simulink model "sampleModel1000"  (R2022a)
settings: Solver=VariableStepAuto  StartTime=0.0  StopTime=10.0  RelTol=1e-3
undefined symbols (not defined in the file): DiscIntNeverNeededParam, magnitude, Newton, Raphson
libraries: simulink x216, slpidlib x76
(part 1 of 10)
settings Model: Creator=TSMC  LastModifiedBy=TSMC

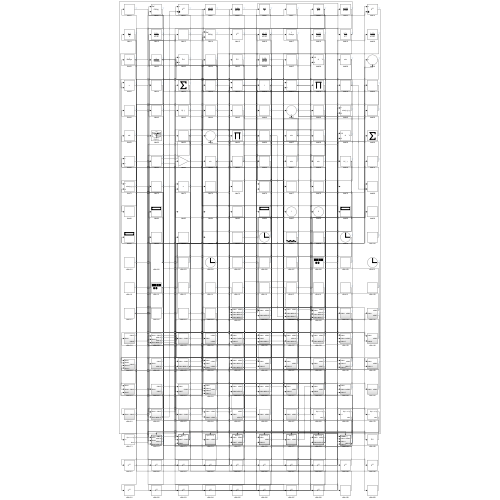
[thumbnail: Simulink's stored preview of the top-level diagram]
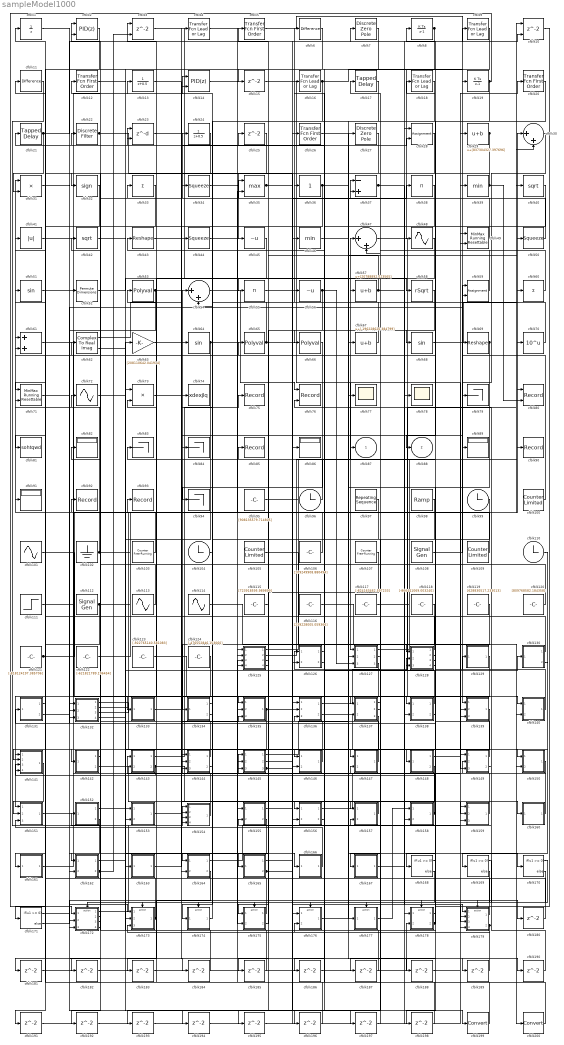
== system sampleModel1000 ==
  cfblk1 : UnitDelay  HasFrameUpgradeWarning=on
  cfblk10 : Delay  ShowEnablePort=on  SampleTime=1
      settings: InputPortMap=u0,e6
  cfblk100 : simulink/Sources/Counter Limited  uplimit=[967.000000]  tsamp=-1
  cfblk101 : Sin  Amplitude=[773063809.845792]  Bias=[655952196.754793]  SampleTime=0
  cfblk102 : Ground
  cfblk103 : simulink/Sources/Counter Free-Running  NumBits=[40.000000]  tsamp=-1
  cfblk{96,99,104,110} (4 alike) : Clock
  cfblk105 : simulink/Sources/Counter Limited  uplimit=[424.000000]  tsamp=-1
  cfblk106 : Constant  Value=[109249908.880494]  SampleTime=1
  cfblk107 : simulink/Sources/Counter Free-Running  NumBits=[50.000000]  tsamp=-1
  cfblk108 : SignalGenerator  WaveForm=sawtooth  Amplitude=[13452965.710921]
  cfblk109 : simulink/Sources/Counter Limited  uplimit=[559.000000]  tsamp=-1
  cfblk11 : simulink/Discrete/Difference  ICPrevInput=0.0  OutMin=[]  OutMax=[]  OutDataTypeStr=Inherit: Inherit via back propagation  OutDataType=fixdt(1, 16)  OutScaling=2^-10  DoSatur=off
  cfblk111 : Step  Time=[14.000000]  Before=[-58060012.443622]  After=[794614404.214897]  SampleTime=0
  cfblk112 : SignalGenerator  WaveForm=sawtooth  Amplitude=[-762282920.604162]  Units=rad/sec
  cfblk113 : Sin  Amplitude=[-356034610.083544]  Bias=[-701710230.192612]  SampleTime=0
  cfblk114 : Sin  Amplitude=[643616227.211529]  Bias=[3557649.516432]  SampleTime=0
  cfblk115 : Constant  Value=[723918595.989899]  SampleTime=1
  cfblk116 : Constant  Value=[239228005.059366]  SampleTime=1
  cfblk117 : Constant  Value=[-824163462.597233]  SampleTime=1
  cfblk118 : Constant  Value=[-866441069.003240]  SampleTime=1
  cfblk119 : Constant  Value=[628830517.233013]  SampleTime=1
  cfblk{5,12,20,26} (4 alike) : simulink/Discrete/Transfer Fcn First Order  PoleZ=0.95  ICPrevOutput=0.0  DoSatur=off
  cfblk120 : Constant  Value=[809768582.184358]  SampleTime=1
  cfblk121 : Constant  Value=[-818124197.385706]  SampleTime=1
  cfblk122 : Constant  Value=[-621821789.196454]  SampleTime=1
  cfblk123 : Constant  Value=[-922765140.581083]  SampleTime=1
  cfblk124 : Constant  Value=[-476552846.153060]  SampleTime=1
  cfblk125 : Subsystem
  cfblk126 : Subsystem
  cfblk127 : Subsystem
  cfblk128 : Subsystem
  cfblk129 : Subsystem
  cfblk13 : DiscreteTransferFcn  SampleTime=1
  cfblk130 : Subsystem
  cfblk131 : Subsystem
  cfblk132 : Subsystem
  cfblk133 : Subsystem
  cfblk134 : Subsystem
  cfblk135 : Subsystem
  cfblk136 : Subsystem
  cfblk137 : Subsystem
  cfblk138 : Subsystem
  cfblk139 : Subsystem
  cfblk14 : slpidlib/PID Controller (2DOF)  Controller=PID  Form=Parallel  TimeDomain=Discrete-time  UseExternalTs=off  SampleTime=1  IntegratorMethod=Forward Euler  FilterMethod=Forward Euler  ControllerParametersSource=internal  P=1  I=1  UseKiTs=off  D=0  N=100  UseFilter=on  b=1  c=1  TunerSelectOption=Transfer Function Based (PID Tuner App)  InitialConditionSource=internal  InitialConditionForIntegrator=0  InitialConditionForFilter=0  DifferentiatorICPrevScaledInput=0  ExternalReset=none  TrackingMode=off  Kt=1  LimitOutput=off  SatLimitsSource=internal  UpperSaturationLimit=inf  LowerSaturationLimit=-inf  LinearizeAsGain=off  AntiWindupMode=none  Kb=1  POutMin=[]  POutMax=[]  IOutMin=[]  IOutMax=[]  DOutMin=[]  DOutMax=[]  NOutMin=[]  NOutMax=[]  bOutMin=[]  bOutMax=[]  cOutMin=[]  cOutMax=[]  SumOutMin=[]  SumOutMax=[]  SaturationOutMin=[]  SaturationOutMax=[]  PParamMin=[]  PParamMax=[]  IParamMin=[]  IParamMax=[]  DParamMin=[]  DParamMax=[]  NParamMin=[]  NParamMax=[]  bParamMin=[]  bParamMax=[]  cParamMin=[]  cParamMax=[]  KbParamMin=[]  KbParamMax=[]  KtParamMin=[]  KtParamMax=[]  KbOutMin=[]  KbOutMax=[]  KtOutMin=[]  KtOutMax=[]  IntegratorOutMin=[]  IntegratorOutMax=[]  FilterOutMin=[]  FilterOutMax=[]  SumI1OutMin=[]  SumI1OutMax=[]  SumI2OutMin=[]  SumI2OutMax=[]  SumI3OutMin=[]  SumI3OutMax=[]  SumI4OutMin=[]  SumI4OutMax=[]  SumDOutMin=[]  SumDOutMax=[]  Sum1OutMin=[]  Sum1OutMax=[]  Sum2OutMin=[]  Sum2OutMax=[]  Sum3OutMin=[]  Sum3OutMax=[]  DifferentiatorOutMin=[]  DifferentiatorOutMax=[]  FilterDiffOutCoefMin=[]  FilterDiffOutCoefMax=[]  ReciprocalOutMin=[]  ReciprocalOutMax=[]  SumDenOutMin=[]  SumDenOutMax=[]  SumNumOutMin=[]  SumNumOutMax=[]  DivideOutMin=[]  DivideOutMax=[]  UdiffTsProdOutMin=[]  UdiffTsProdOutMax=[]  NTsProdOutMin=[]  NTsProdOutMax=[]  UintegralTsProdOutMin=[]  UintegralTsProdOutMax=[]  UngainTsProdOutMin=[]  UngainTsProdOutMax=[]  IntegratorContinuousStateAttributes=''  IntegratorStateMustResolveToSignalObject=off  IntegratorRTWStateStorageClass=Auto  FilterContinuousStateAttributes=''  FilterStateMustResolveToSignalObject=off  FilterRTWStateStorageClass=Auto  ParallelPVariant=InternalParameters  IdealPVariant=Disabled  IVariant=InternalParameters  DVariant=InternalParameters  bVariant=InternalParameters  cVariant=InternalParameters  IntegratorVariant=Discrete  SatVariant=Disabled  AWVariant=Passthrough  PCopyVariant=Disabled  TRVariant=Disabled  FdbkBlocksVariant=Forward  IdealPFdbkVariant=Disabled  SatFdbkVariant=Disabled  DerivativeFilterVariant=ForwardEulerFilter  NVariant=InternalParameters  NCopyVariant=Disabled  FilterICVariant=InternalICsFilter  IntegratorICVariant=InternalICs  ExternalResetVariant=Disabled  TRSumVariant=Passthrough  SumFdbkVariant=Disabled  SumVariant=Sum_PID  TsampFilterVariant=InternalTs  TsampNgainVariant=Passthrough  TsampIntegralVariant=Passthrough  ExternalSaturationOutDataTypeStr=Inherit: Same as second input
      settings: SourceProductBaseCode=SL
  cfblk140 : Subsystem
  cfblk141 : Subsystem
  cfblk142 : Subsystem
  cfblk143 : Subsystem
  cfblk144 : Subsystem
  cfblk145 : Subsystem
  cfblk146 : Subsystem
  cfblk147 : Subsystem
  cfblk148 : Subsystem
  cfblk149 : Subsystem
  cfblk{15,25,180..198} (21 alike) : Delay  SampleTime=1
  cfblk150 : Subsystem
  cfblk151 : Subsystem
  cfblk152 : Subsystem
  cfblk153 : Subsystem
  cfblk154 : Subsystem
  cfblk155 : Subsystem
  cfblk156 : Subsystem
  cfblk157 : Subsystem
  cfblk158 : Subsystem
  cfblk159 : Subsystem
  cfblk{4,9,16,18} (4 alike) : simulink/Discrete/Transfer Fcn Lead or Lag  PoleZ=0.95  ZeroZ=0.75  ICPrevOutput=0.0  ICPrevInput=0.0  DoSatur=off
      settings: SourceProductBaseCode=SL
  cfblk160 : Subsystem
  cfblk161 : Subsystem
  cfblk162 : Subsystem
  cfblk163 : Subsystem
  cfblk164 : Subsystem
  cfblk165 : Subsystem
  cfblk166 : Subsystem
  cfblk167 : Subsystem
  cfblk{168..171} (4 alike) : If  IfExpression=u1 >= 0  SampleTime=1
  cfblk17 : simulink/Discrete/Tapped Delay  vinit=0.0  samptime=-1  NumDelays=1  DelayOrder=Oldest  includeCurrent=off
  cfblk172 : Subsystem  TreatAsAtomicUnit=on
  cfblk173 : Subsystem  TreatAsAtomicUnit=on
  cfblk174 : Subsystem  TreatAsAtomicUnit=on
  cfblk175 : Subsystem  TreatAsAtomicUnit=on
  cfblk176 : Subsystem  TreatAsAtomicUnit=on
  cfblk177 : Subsystem  TreatAsAtomicUnit=on
  cfblk178 : Subsystem  TreatAsAtomicUnit=on
  cfblk179 : Subsystem  TreatAsAtomicUnit=on
  cfblk19 : DiscreteIntegrator  ICPrevOutput=DiscIntNeverNeededParam  ICPrevScaledInput=DiscIntNeverNeededParam
  cfblk199 : DataTypeConversion  SaturateOnIntegerOverflow=off  RndMeth=Floor
  cfblk2 : slpidlib/PID Controller (2DOF)  Controller=PID  Form=Parallel  TimeDomain=Discrete-time  UseExternalTs=off  SampleTime=1  IntegratorMethod=Forward Euler  FilterMethod=Forward Euler  ControllerParametersSource=internal  P=1  I=1  UseKiTs=off  D=0  N=100  UseFilter=on  b=1  c=1  TunerSelectOption=Transfer Function Based (PID Tuner App)  InitialConditionSource=internal  InitialConditionForIntegrator=0  InitialConditionForFilter=0  DifferentiatorICPrevScaledInput=0  ExternalReset=none  TrackingMode=off  Kt=1  LimitOutput=off  SatLimitsSource=internal  UpperSaturationLimit=inf  LowerSaturationLimit=-inf  LinearizeAsGain=off  AntiWindupMode=none  Kb=1  POutMin=[]  POutMax=[]  IOutMin=[]  IOutMax=[]  DOutMin=[]  DOutMax=[]  NOutMin=[]  NOutMax=[]  bOutMin=[]  bOutMax=[]  cOutMin=[]  cOutMax=[]  SumOutMin=[]  SumOutMax=[]  SaturationOutMin=[]  SaturationOutMax=[]  PParamMin=[]  PParamMax=[]  IParamMin=[]  IParamMax=[]  DParamMin=[]  DParamMax=[]  NParamMin=[]  NParamMax=[]  bParamMin=[]  bParamMax=[]  cParamMin=[]  cParamMax=[]  KbParamMin=[]  KbParamMax=[]  KtParamMin=[]  KtParamMax=[]  KbOutMin=[]  KbOutMax=[]  KtOutMin=[]  KtOutMax=[]  IntegratorOutMin=[]  IntegratorOutMax=[]  FilterOutMin=[]  FilterOutMax=[]  SumI1OutMin=[]  SumI1OutMax=[]  SumI2OutMin=[]  SumI2OutMax=[]  SumI3OutMin=[]  SumI3OutMax=[]  SumI4OutMin=[]  SumI4OutMax=[]  SumDOutMin=[]  SumDOutMax=[]  Sum1OutMin=[]  Sum1OutMax=[]  Sum2OutMin=[]  Sum2OutMax=[]  Sum3OutMin=[]  Sum3OutMax=[]  DifferentiatorOutMin=[]  DifferentiatorOutMax=[]  FilterDiffOutCoefMin=[]  FilterDiffOutCoefMax=[]  ReciprocalOutMin=[]  ReciprocalOutMax=[]  SumDenOutMin=[]  SumDenOutMax=[]  SumNumOutMin=[]  SumNumOutMax=[]  DivideOutMin=[]  DivideOutMax=[]  UdiffTsProdOutMin=[]  UdiffTsProdOutMax=[]  NTsProdOutMin=[]  NTsProdOutMax=[]  UintegralTsProdOutMin=[]  UintegralTsProdOutMax=[]  UngainTsProdOutMin=[]  UngainTsProdOutMax=[]  IntegratorContinuousStateAttributes=''  IntegratorStateMustResolveToSignalObject=off  IntegratorRTWStateStorageClass=Auto  FilterContinuousStateAttributes=''  FilterStateMustResolveToSignalObject=off  FilterRTWStateStorageClass=Auto  ParallelPVariant=InternalParameters  IdealPVariant=Disabled  IVariant=InternalParameters  DVariant=InternalParameters  bVariant=InternalParameters  cVariant=InternalParameters  IntegratorVariant=Discrete  SatVariant=Disabled  AWVariant=Passthrough  PCopyVariant=Disabled  TRVariant=Disabled  FdbkBlocksVariant=Forward  IdealPFdbkVariant=Disabled  SatFdbkVariant=Disabled  DerivativeFilterVariant=ForwardEulerFilter  NVariant=InternalParameters  NCopyVariant=Disabled  FilterICVariant=InternalICsFilter  IntegratorICVariant=InternalICs  ExternalResetVariant=Disabled  TRSumVariant=Passthrough  SumFdbkVariant=Disabled  SumVariant=Sum_PID  TsampFilterVariant=InternalTs  TsampNgainVariant=Passthrough  TsampIntegralVariant=Passthrough  ExternalSaturationOutDataTypeStr=Inherit: Same as second input
      settings: SourceProductBaseCode=SL
  cfblk200 : DataTypeConversion  SaturateOnIntegerOverflow=off  RndMeth=Floor
  cfblk21 : simulink/Discrete/Tapped Delay  vinit=0.0  samptime=-1  NumDelays=1  DelayOrder=Oldest  includeCurrent=off
  cfblk22 : DiscreteFilter  SampleTime=1
  cfblk23 : Delay  DelayLengthSource=Input port  SampleTime=1
      settings: InputPortMap=u0,p1
  cfblk24 : DiscreteTransferFcn  SampleTime=1
  cfblk27 : DiscreteZeroPole  Poles=[0 0.5]  Gain=1
  cfblk28 : Assignment  DiagnosticForDimensions=Warning  IndexOptions=Index vector (dialog)  Indices=1  OutputSizes=1
  cfblk29 : Bias  Bias=[837304327.397696]  SaturateOnIntegerOverflow=off
  cfblk3 : Delay  ShowEnablePort=on  SampleTime=1
      settings: InputPortMap=u0,e6
  cfblk30 : Sum  Inputs=|++
  cfblk31 : Product
  cfblk32 : Signum
  cfblk33 : Sum  Inputs=+
  cfblk34 : Squeeze
  cfblk35 : MinMax  Function=max  Inputs=2
  cfblk36 : simulink/Math Operations/Slider Gain  gain=1  low=0  high=2
  cfblk37 : Sum  Inputs=-+
  cfblk38 : Product  Inputs=*
  cfblk39 : MinMax
  cfblk40 : Sqrt
  cfblk41 : Abs  SaturateOnIntegerOverflow=off
  cfblk42 : Sqrt
  cfblk43 : Reshape
  cfblk44 : Squeeze
  cfblk45 : UnaryMinus
  cfblk46 : MinMax
  cfblk47 : Sum  Inputs=|++
  cfblk48 : Sin  TimeSource=Use external signal  SampleTime=0
  cfblk49 : simulink/Math Operations/MinMax Running Resettable  Function=min  vinit=0.0
  cfblk50 : Squeeze
  cfblk51 : Trigonometry
  cfblk52 : PermuteDimensions
  cfblk53 : Polyval  Coefs=[ +2.081618890e-019, -1.441693666e-014, +4.719686976e-010, -8.536869453e-006, +1.621573104e-001, -8.087801117e+001 ]
  cfblk54 : Sum  Inputs=|++
  cfblk55 : Product  Inputs=*
  cfblk56 : UnaryMinus
  cfblk57 : Bias  Bias=[20788892.023565]  SaturateOnIntegerOverflow=off
  cfblk58 : Sqrt  Operator=rSqrt  AlgorithmType=Newton-Raphson
  cfblk59 : Assignment  DiagnosticForDimensions=Warning  IndexOptions=Index vector (dialog)  Indices=1  OutputSizes=1
  cfblk6 : simulink/Discrete/Difference  ICPrevInput=0.0  OutMin=[]  OutMax=[]  OutDataTypeStr=Inherit: Inherit via back propagation  OutDataType=fixdt(1, 16)  OutScaling=2^-10  DoSatur=off
  cfblk60 : Sum  Inputs=+
  cfblk61 : Sum
  cfblk62 : ComplexToRealImag
  cfblk63 : Gain  Gain=[208110642.041914]
  cfblk64 : Trigonometry
  cfblk65 : Polyval  Coefs=[ +2.081618890e-019, -1.441693666e-014, +4.719686976e-010, -8.536869453e-006, +1.621573104e-001, -8.087801117e+001 ]
  cfblk66 : Polyval  Coefs=[ +2.081618890e-019, -1.441693666e-014, +4.719686976e-010, -8.536869453e-006, +1.621573104e-001, -8.087801117e+001 ]
  cfblk67 : Bias  Bias=[-196228620.384799]  SaturateOnIntegerOverflow=off
  cfblk68 : Trigonometry
  cfblk69 : Reshape
  cfblk7 : DiscreteZeroPole  Poles=[0 0.5]  Gain=1
  cfblk70 : Math  Operator=10^u
  cfblk71 : simulink/Math Operations/MinMax Running Resettable  Function=min  vinit=0.0
  cfblk72 : Sin  TimeSource=Use external signal  SampleTime=0
  cfblk73 : Product  Inputs=**
  cfblk74 : ToWorkspace  VariableName=xdexjlq  SaveFormat=Timeseries  SampleTime=-1
  cfblk75 : Record  FileSettingsInternal="{\"entries\":[{\"content\":{\"excelSettings\":{\"content\":{},\"type\":\"Streamout.ExcelSettings\"}},\"type\":\"Streamout.FileSettingStorage\",\"uuid\":\"93119369-c950-46ca-a22c-1d32b41a04c2\"}],\"packageUris\":[\"http://schema.mathworks.com/mf0/streamout_blocks/R2020a\"],\"version\":\"1.0\"}"  SignalsInternal="{\"entries\":[{\"content\":{\"signals\":[]},\"type\":\"RecordBlkView.InputSignals\",\"uuid\":\"8868a1fd-9bce-4a45-8f3b-298cfc814564\"}],\"packageUris\":[\"http://schema.mathworks.com/mf0/streamout_blocks/R2020a\"],\"version\":\"1.0\"}"  VisualizationBindings="{\"sparklinesplugin\":{\"info\":[{\"bindingParametersList\":[],\"subplotID\":1}]}}"
  cfblk76 : Record  FileSettingsInternal="{\"entries\":[{\"content\":{\"excelSettings\":{\"content\":{},\"type\":\"Streamout.ExcelSettings\"}},\"type\":\"Streamout.FileSettingStorage\",\"uuid\":\"a03253ba-281f-4ced-abad-5bfd2517a59d\"}],\"packageUris\":[\"http://schema.mathworks.com/mf0/streamout_blocks/R2020a\"],\"version\":\"1.0\"}"  Layout=[1 1]  SignalsInternal="{\"entries\":[{\"content\":{\"signals\":[{\"content\":{\"blockPath\":[\"sampleModel93/cfblk76\"],\"channel\":[],\"dimensions\":[1],\"domain\":\"sampleModel93/cfblk76\",\"lineColor\":\"#a2142f\",\"plots\":[1],\"port\":1,\"sid\":[],\"signalID\":93159,\"signalName\":\"XY Graph:1\"},\"type\":\"RecordBlkView.Signal\",\"uuid\":\"edc37d75-abdc-4082-bde9-98d4d700ed05\"},{\"content\":{\"blockPath\":[\"sampleModel93/cfblk76\"],\"channel\":[],\"dimensions\":[1],\"domain\":\"sampleModel93/cfblk76\",\"lineColor\":\"#139fff\",\"plots\":[1],\"port\":2,\"sid\":[],\"signalID\":93162,\"signalName\":\"XY Graph:2\"},\"type\":\"RecordBlkView.Signal\",\"uuid\":\"72f55811-d401-47ba-bcf8-176263eeb075\"}]},\"type\":\"RecordBlkView.InputSignals\",\"uuid\":\"5a81d43f-68da-4077-b013-bac875f31b79\"}],\"packageUris\":[\"http://schema.mathworks.com/mf0/streamout_blocks/R2020a\"],\"version\":\"1.0\"}"  VisualizationBindings="{\"xyplotplugin\":{\"info\":[{\"series\":[{\"bindingParametersList\":[{\"parameter\":\"X-Axis\",\"signalID\":93159,\"signalName\":\"XY Graph:1\"},{\"parameter\":\"Y-Axis\",\"signalID\":93162,\"signalName\":\"XY Graph:2\"}],\"seriesID\":38366}],\"subplotID\":1}]}}"  CompatibilityTag=XY
  cfblk77 : Scope
  cfblk78 : Scope
  cfblk{79,83..84,94} (4 alike) : Terminator
  cfblk8 : DiscreteIntegrator  ICPrevOutput=DiscIntNeverNeededParam  ICPrevScaledInput=DiscIntNeverNeededParam
  cfblk80 : Record  FileSettingsInternal="{\"entries\":[{\"content\":{\"excelSettings\":{\"content\":{},\"type\":\"Streamout.ExcelSettings\"}},\"type\":\"Streamout.FileSettingStorage\",\"uuid\":\"2507d3ea-2c9f-47b8-9c6a-10834b2444f5\"}],\"packageUris\":[\"http://schema.mathworks.com/mf0/streamout_blocks/R2020a\"],\"version\":\"1.0\"}"  Layout=[1 1]  SignalsInternal="{\"entries\":[{\"content\":{\"signals\":[{\"content\":{\"blockPath\":[\"sampleModel93/cfblk80\"],\"channel\":[],\"dimensions\":[1],\"domain\":\"sampleModel93/cfblk80\",\"lineColor\":\"#a2142f\",\"plots\":[1],\"port\":1,\"sid\":[],\"signalID\":93167,\"signalName\":\"XY Graph:1\"},\"type\":\"RecordBlkView.Signal\",\"uuid\":\"5814ea94-654b-43ff-b425-7d5855ec870a\"},{\"content\":{\"blockPath\":[\"sampleModel93/cfblk80\"],\"channel\":[],\"dimensions\":[1],\"domain\":\"sampleModel93/cfblk80\",\"lineColor\":\"#139fff\",\"plots\":[1],\"port\":2,\"sid\":[],\"signalID\":93170,\"signalName\":\"XY Graph:2\"},\"type\":\"RecordBlkView.Signal\",\"uuid\":\"afd25cc8-4550-43db-8d86-e57050363295\"}]},\"type\":\"RecordBlkView.InputSignals\",\"uuid\":\"2447f943-610b-4a01-b7b9-18fff63071f0\"}],\"packageUris\":[\"http://schema.mathworks.com/mf0/streamout_blocks/R2020a\"],\"version\":\"1.0\"}"  VisualizationBindings="{\"xyplotplugin\":{\"info\":[{\"series\":[{\"bindingParametersList\":[{\"parameter\":\"X-Axis\",\"signalID\":93167,\"signalName\":\"XY Graph:1\"},{\"parameter\":\"Y-Axis\",\"signalID\":93170,\"signalName\":\"XY Graph:2\"}],\"seriesID\":65284}],\"subplotID\":1}]}}"  CompatibilityTag=XY
  cfblk81 : ToWorkspace  VariableName=sohtqwd  SaveFormat=Timeseries  SampleTime=-1
  cfblk{82,86,89,91} (4 alike) : Display
  cfblk85 : Record  FileSettingsInternal="{\"entries\":[{\"content\":{\"excelSettings\":{\"content\":{},\"type\":\"Streamout.ExcelSettings\"}},\"type\":\"Streamout.FileSettingStorage\",\"uuid\":\"56e11c23-7fef-42fd-95e6-2b1f2738764b\"}],\"packageUris\":[\"http://schema.mathworks.com/mf0/streamout_blocks/R2020a\"],\"version\":\"1.0\"}"  SignalsInternal="{\"entries\":[{\"content\":{\"signals\":[]},\"type\":\"RecordBlkView.InputSignals\",\"uuid\":\"a01aa0e3-d666-47db-b4e9-c308bb60c8cd\"}],\"packageUris\":[\"http://schema.mathworks.com/mf0/streamout_blocks/R2020a\"],\"version\":\"1.0\"}"  VisualizationBindings="{\"sparklinesplugin\":{\"info\":[{\"bindingParametersList\":[],\"subplotID\":1}]}}"
  cfblk90 : Record  FileSettingsInternal="{\"entries\":[{\"content\":{\"excelSettings\":{\"content\":{},\"type\":\"Streamout.ExcelSettings\"}},\"type\":\"Streamout.FileSettingStorage\",\"uuid\":\"6dada1e4-55e1-4f5a-970b-daff20d2999b\"}],\"packageUris\":[\"http://schema.mathworks.com/mf0/streamout_blocks/R2020a\"],\"version\":\"1.0\"}"  SignalsInternal="{\"entries\":[{\"content\":{\"signals\":[]},\"type\":\"RecordBlkView.InputSignals\",\"uuid\":\"89ee935f-d475-4a10-a7b9-b698c62ff7ff\"}],\"packageUris\":[\"http://schema.mathworks.com/mf0/streamout_blocks/R2020a\"],\"version\":\"1.0\"}"  VisualizationBindings="{\"sparklinesplugin\":{\"info\":[{\"bindingParametersList\":[],\"subplotID\":1}]}}"
  cfblk92 : Record  FileSettingsInternal="{\"entries\":[{\"content\":{\"excelSettings\":{\"content\":{},\"type\":\"Streamout.ExcelSettings\"}},\"type\":\"Streamout.FileSettingStorage\",\"uuid\":\"1238a7f8-d0eb-4180-8fbc-9d1406293420\"}],\"packageUris\":[\"http://schema.mathworks.com/mf0/streamout_blocks/R2020a\"],\"version\":\"1.0\"}"  SignalsInternal="{\"entries\":[{\"content\":{\"signals\":[]},\"type\":\"RecordBlkView.InputSignals\",\"uuid\":\"67d9e696-d9a1-4a8c-bdff-202bc9e338b2\"}],\"packageUris\":[\"http://schema.mathworks.com/mf0/streamout_blocks/R2020a\"],\"version\":\"1.0\"}"  VisualizationBindings="{\"sparklinesplugin\":{\"info\":[{\"bindingParametersList\":[],\"subplotID\":1}]}}"
  cfblk93 : Record  FileSettingsInternal="{\"entries\":[{\"content\":{\"excelSettings\":{\"content\":{},\"type\":\"Streamout.ExcelSettings\"}},\"type\":\"Streamout.FileSettingStorage\",\"uuid\":\"aa34f245-15e1-43bc-9a71-911d6946ae5d\"}],\"packageUris\":[\"http://schema.mathworks.com/mf0/streamout_blocks/R2020a\"],\"version\":\"1.0\"}"  SignalsInternal="{\"entries\":[{\"content\":{\"signals\":[]},\"type\":\"RecordBlkView.InputSignals\",\"uuid\":\"ca37f52f-a70f-4701-97d8-d5f8771f9d64\"}],\"packageUris\":[\"http://schema.mathworks.com/mf0/streamout_blocks/R2020a\"],\"version\":\"1.0\"}"  VisualizationBindings="{\"sparklinesplugin\":{\"info\":[{\"bindingParametersList\":[],\"subplotID\":1}]}}"
  cfblk95 : Constant  Value=[908135579.714805]  SampleTime=1
  cfblk97 : simulink/Sources/Repeating Sequence  rep_seq_t=[0 2]  rep_seq_y=[-687576342.069887, -842837087.753460]
  cfblk98 : simulink/Sources/Ramp  slope=[9655.940624]  start=[7.462579]  InitialOutput=[164286.432443]
  cfblk87 : Outport
  cfblk88 : Outport  Port=2
  wires:
  cfblk124/1 -> cfblk151/1(cfblk1)
  cfblk66/1 -> cfblk174/1(cfblk1)
  cfblk54/1 -> cfblk76/1
  cfblk154/1(cfblk2) -> cfblk54/1
  cfblk58/1 -> cfblk135/1(cfblk1)
  cfblk3/1 -> cfblk86/1
  cfblk6/1 -> cfblk15/1
  cfblk11/1 -> cfblk154/1(cfblk1)
  cfblk151/1(cfblk2) -> cfblk14/1
  cfblk5/1 -> cfblk139/1(cfblk1)
  cfblk70/1 -> cfblk21/1
  cfblk47/1 -> cfblk140/1(cfblk1)
  cfblk177/1(cfblk2) -> cfblk158/1(cfblk1)
  cfblk108/1 -> cfblk59/1
  cfblk49/1 -> cfblk24/1
  cfblk25/1 -> cfblk45/1
  cfblk125/1(cfblk2) -> cfblk47/1
  cfblk30/1 -> cfblk79/1
  cfblk41/1 -> cfblk13/1
  cfblk157/1(cfblk2) -> cfblk154/2(cfblk15)
  cfblk9/1 -> cfblk48/1
  cfblk143/1(cfblk2) -> cfblk75/1
  cfblk117/1 -> cfblk30/1
  cfblk61/1 -> cfblk138/1(cfblk1)
  cfblk153/1(cfblk2) -> cfblk166/1(cfblk1)
  cfblk118/1 -> cfblk134/1(cfblk1)
  cfblk109/1 -> cfblk31/1
  cfblk27/1 -> cfblk141/1(cfblk1)
  cfblk56/1 -> cfblk127/3(cfblk15), cfblk195/1
  cfblk15/1 -> cfblk127/1(cfblk1)
  cfblk134/1(cfblk2) -> cfblk142/1(cfblk1)
  cfblk104/1 -> cfblk14/2
  cfblk67/1 -> cfblk6/1
  cfblk123/1 -> cfblk138/2(cfblk11)
  cfblk23/1 -> cfblk144/1(cfblk1)
  cfblk173/1(cfblk2) -> cfblk91/1, cfblk82/1
  cfblk110/1 -> cfblk169/1
  cfblk64/1 -> cfblk153/2(cfblk7), cfblk156/2(cfblk12)
  cfblk121/1 -> cfblk154/3(cfblk16), cfblk4/1
  cfblk161/1(cfblk2) -> cfblk29/1
  cfblk48/1 -> cfblk55/1
  cfblk55/1 -> cfblk177/1(cfblk1)
  cfblk146/1(cfblk2) -> cfblk42/1
  cfblk37/1 -> cfblk78/1, cfblk10/2
  cfblk138/1(cfblk2) -> cfblk36/1
  cfblk69/1 -> cfblk168/1, cfblk137/2(cfblk13)
  cfblk21/1 -> cfblk31/2, cfblk9/1
  cfblk39/1 -> cfblk32/1, cfblk80/2
  cfblk65/1 -> cfblk149/1(cfblk1), cfblk23/2
  cfblk10/1 -> cfblk155/2(cfblk9)
  cfblk133/1(cfblk2) -> cfblk136/2(cfblk9)
  cfblk68/1 -> cfblk60/1
  cfblk132/1(cfblk2) -> cfblk147/1(cfblk1)
  cfblk60/1 -> cfblk17/1
  cfblk141/1(cfblk2) -> cfblk151/2(cfblk6)
  cfblk148/1(cfblk2) -> cfblk20/1
  cfblk127/1(cfblk2) -> cfblk39/1
  cfblk107/1 -> cfblk175/1(cfblk1)
  cfblk136/1(cfblk2) -> cfblk30/2
  cfblk150/1(cfblk2) -> cfblk149/2(cfblk15)
  cfblk126/2(cfblk12) -> cfblk43/1
  cfblk156/1(cfblk2) -> cfblk28/1
  cfblk53/1 -> cfblk87/1, cfblk132/3(cfblk14)
  cfblk100/1 -> cfblk69/1
  cfblk143/2(cfblk13) -> cfblk160/1(cfblk1), cfblk141/4(cfblk11), cfblk135/3(cfblk16)
  cfblk172/1(cfblk2) -> cfblk28/2
  cfblk44/1 -> cfblk140/2(cfblk8)
  cfblk131/1(cfblk2) -> cfblk51/1
  cfblk138/2(cfblk12) -> cfblk62/1
  cfblk137/1(cfblk2) -> cfblk157/1(cfblk1)
  cfblk51/1 -> cfblk52/1
  cfblk19/1 -> cfblk172/1(cfblk1), cfblk127/2(cfblk14)
  cfblk130/1(cfblk2) -> cfblk18/1
  cfblk120/1 -> cfblk33/1
  cfblk115/1 -> cfblk165/1(cfblk1)
  cfblk174/1(cfblk2) -> cfblk54/2
  cfblk145/1(cfblk2) -> cfblk27/1
  cfblk160/1(cfblk2) -> cfblk47/2
  cfblk103/1 -> cfblk93/1
  cfblk7/1 -> cfblk172/2(cfblk8)
  cfblk8/1 -> cfblk146/1(cfblk1), cfblk173/2(cfblk7)
  cfblk131/2(cfblk8) -> cfblk59/2
  cfblk144/1(cfblk2) -> cfblk22/1
  cfblk35/1 -> cfblk46/1, cfblk197/1
  cfblk130/2(cfblk7) -> cfblk150/1(cfblk1)
  cfblk179/1(cfblk2) -> cfblk5/1
  cfblk22/1 -> cfblk56/1, cfblk196/1
  cfblk144/2(cfblk9) -> cfblk74/1
  cfblk142/1(cfblk2) -> cfblk12/1
  cfblk62/1 -> cfblk44/1
  cfblk164/1(cfblk2) -> cfblk49/1
  cfblk73/1 -> cfblk159/2(cfblk14)
  cfblk179/2(cfblk13) -> cfblk129/1(cfblk1), cfblk176/2(cfblk16), cfblk157/2(cfblk10), cfblk173/3(cfblk8)
  cfblk116/1 -> cfblk139/2(cfblk14)
  cfblk17/1 -> cfblk156/1(cfblk1)
  cfblk42/1 -> cfblk139/3(cfblk15)
  cfblk176/1(cfblk2) -> cfblk50/1
  cfblk57/1 -> cfblk35/1, cfblk179/3(cfblk11)
  cfblk149/1(cfblk2) -> cfblk8/1
  cfblk158/1(cfblk2) -> cfblk16/1, cfblk141/3(cfblk10)
  cfblk155/1(cfblk2) -> cfblk26/1
  cfblk101/1 -> cfblk146/2(cfblk16)
  cfblk152/2(cfblk7) -> cfblk172/3(cfblk9)
  cfblk97/1 -> cfblk164/1(cfblk1)
  cfblk33/1 -> cfblk171/1
  cfblk40/1 -> cfblk68/1
  cfblk111/1 -> cfblk35/2
  cfblk114/1 -> cfblk128/1(cfblk1)
  cfblk132/2(cfblk15) -> cfblk150/2(cfblk11)
  cfblk59/1 -> cfblk34/1
  cfblk159/1(cfblk2) -> cfblk145/1(cfblk1)
  cfblk16/1 -> cfblk19/1, cfblk125/4(cfblk14)
  cfblk4/1 -> cfblk125/1(cfblk1)
  cfblk156/2(cfblk13) -> cfblk25/1
  cfblk125/2(cfblk15) -> cfblk77/1
  cfblk136/2(cfblk11) -> cfblk148/1(cfblk1)
  cfblk128/1(cfblk2) -> cfblk11/1
  cfblk162/1(cfblk2) -> cfblk63/1
  cfblk31/1 -> cfblk173/1(cfblk1)
  cfblk128/2(cfblk15) -> cfblk57/1
  cfblk62/2 -> cfblk163/1(cfblk1)
  cfblk175/1(cfblk2) -> cfblk73/2
  cfblk95/1 -> cfblk70/1
  cfblk125/3(cfblk16) -> cfblk85/1
  cfblk142/2(cfblk14) -> cfblk154/4(cfblk17)
  cfblk20/1 -> cfblk88/1
  cfblk122/1 -> cfblk80/1
  cfblk163/1(cfblk2) -> cfblk128/2(cfblk13)
  cfblk72/1 -> cfblk164/2(cfblk8)
  cfblk106/1 -> cfblk3/1
  cfblk155/2(cfblk10) -> cfblk162/1(cfblk1)
  cfblk43/1 -> cfblk149/3(cfblk16)
  cfblk132/3(cfblk16) -> cfblk10/1
  cfblk38/1 -> cfblk66/1
  cfblk36/1 -> cfblk71/1, cfblk179/2(cfblk10)
  cfblk13/1 -> cfblk89/1
  cfblk145/2(cfblk14) -> cfblk7/1
  cfblk165/1(cfblk2) -> cfblk179/1(cfblk1)
  cfblk134/2(cfblk8) -> cfblk61/1
  cfblk28/1 -> cfblk81/1
  cfblk140/1(cfblk2) -> cfblk83/1
  cfblk167/1(cfblk2) -> cfblk90/1
  cfblk128/4(cfblk17) -> cfblk65/1
  cfblk98/1 -> cfblk135/2(cfblk15)
  cfblk125/4(cfblk17) -> cfblk23/1
  cfblk145/3(cfblk15) -> cfblk130/1(cfblk1), cfblk61/2
  cfblk99/1 -> cfblk167/1(cfblk1)
  cfblk162/2(cfblk15) -> cfblk152/1(cfblk1), cfblk3/2
  cfblk45/1 -> cfblk133/1(cfblk1)
  cfblk34/1 -> cfblk137/1(cfblk1)
  cfblk52/1 -> cfblk58/1
  cfblk18/1 -> cfblk94/1
  cfblk149/2(cfblk17) -> cfblk76/2
  cfblk32/1 -> cfblk162/2(cfblk14)
  cfblk178/2(cfblk10) -> cfblk37/1, cfblk131/1(cfblk1)
  cfblk96/1 -> cfblk84/1
  cfblk113/1 -> cfblk2/1
  cfblk148/2(cfblk7) -> cfblk175/2(cfblk7)
  cfblk147/1(cfblk2) -> cfblk64/1
  cfblk112/1 -> cfblk161/1(cfblk1), cfblk67/1
  cfblk46/1 -> cfblk170/1
  cfblk175/2(cfblk8) -> cfblk143/1(cfblk1)
  cfblk135/1(cfblk2) -> cfblk176/1(cfblk1), cfblk192/1
  cfblk166/1(cfblk2) -> cfblk151/3(cfblk7)
  cfblk119/1 -> cfblk125/2(cfblk12)
  cfblk172/3(cfblk11) -> cfblk72/1
  cfblk172/4(cfblk12) -> cfblk71/2
  cfblk12/1 -> cfblk144/2(cfblk7)
  cfblk127/3(cfblk17) -> cfblk143/2(cfblk12)
  cfblk102/1 -> cfblk41/1, cfblk40/1
  cfblk50/1 -> cfblk2/2
  cfblk137/2(cfblk14) -> cfblk126/1(cfblk1)
  cfblk165/2(cfblk14) -> cfblk38/1, cfblk92/1
  cfblk137/3(cfblk15) -> cfblk141/2(cfblk9)
  cfblk29/1 -> cfblk144/3(cfblk8), cfblk126/2(cfblk11)
  cfblk132/4(cfblk17) -> cfblk128/3(cfblk14)
  cfblk168/1 -> cfblk172/Action
  cfblk168/2 -> cfblk173/Action
  cfblk169/1 -> cfblk174/Action
  cfblk169/2 -> cfblk175/Action
  cfblk170/1 -> cfblk176/Action
  cfblk170/2 -> cfblk177/Action
  cfblk171/1 -> cfblk178/Action
  cfblk171/2 -> cfblk179/Action
  cfblk14/1 -> cfblk180/1
  cfblk180/1 -> cfblk153/1(cfblk1)
  cfblk172/2(cfblk10) -> cfblk181/1
  cfblk181/1 -> cfblk145/2(cfblk12)
  cfblk24/1 -> cfblk182/1
  cfblk182/1 -> cfblk49/2
  cfblk164/2(cfblk9) -> cfblk183/1
  cfblk183/1 -> cfblk145/3(cfblk13)
  cfblk71/1 -> cfblk184/1
  cfblk184/1 -> cfblk132/1(cfblk1)
  cfblk139/1(cfblk2) -> cfblk185/1
  cfblk185/1 -> cfblk73/1
  cfblk129/1(cfblk2) -> cfblk186/1
  cfblk186/1 -> cfblk178/2(cfblk9)
  cfblk178/1(cfblk2) -> cfblk187/1
  cfblk187/1 -> cfblk132/2(cfblk13)
  cfblk26/1 -> cfblk188/1
  cfblk188/1 -> cfblk159/1(cfblk1)
  cfblk63/1 -> cfblk189/1
  cfblk189/1 -> cfblk37/2
  cfblk152/1(cfblk2) -> cfblk190/1
  cfblk190/1 -> cfblk155/1(cfblk1)
  cfblk2/1 -> cfblk191/1
  cfblk191/1 -> cfblk159/3(cfblk15)
  cfblk192/1 -> cfblk179/4(cfblk12)
  cfblk126/1(cfblk2) -> cfblk193/1
  cfblk193/1 -> cfblk178/1(cfblk1)
  cfblk127/2(cfblk16) -> cfblk194/1
  cfblk194/1 -> cfblk158/2(cfblk8)
  cfblk195/1 -> cfblk136/1(cfblk1)
  cfblk196/1 -> cfblk125/3(cfblk13)
  cfblk197/1 -> cfblk147/2(cfblk12)
  cfblk128/3(cfblk16) -> cfblk198/1
  cfblk198/1 -> cfblk136/3(cfblk10)
  cfblk1/1 -> cfblk199/1
  cfblk199/1 -> cfblk53/1
  cfblk105/1 -> cfblk200/1
  cfblk200/1 -> cfblk1/1

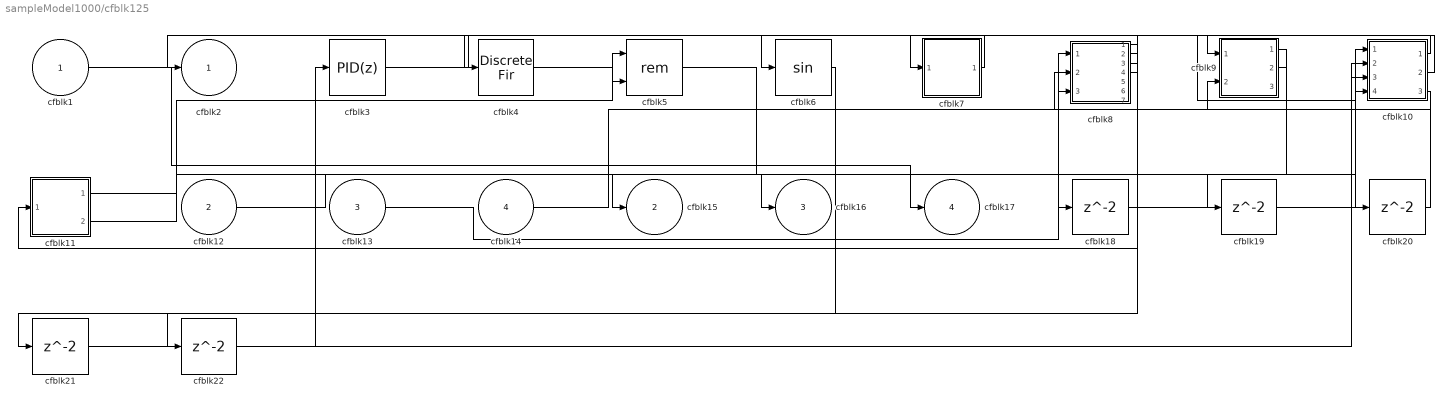
== system sampleModel1000/cfblk125 ==
  cfblk1 : Inport
  cfblk12 : Inport  Port=2
  cfblk13 : Inport  Port=3
  cfblk14 : Inport  Port=4
  cfblk10 : Subsystem
  cfblk11 : Subsystem
  cfblk{18..22} (5 alike) : Delay  SampleTime=1
  cfblk3 : slpidlib/PID Controller  Controller=PID  Form=Parallel  TimeDomain=Discrete-time  UseExternalTs=off  SampleTime=1  IntegratorMethod=Forward Euler  FilterMethod=Forward Euler  ControllerParametersSource=internal  P=1  I=1  UseKiTs=off  D=0  N=100  UseFilter=on  TunerSelectOption=Transfer Function Based (PID Tuner App)  InitialConditionSource=internal  InitialConditionForIntegrator=0  InitialConditionForFilter=0  DifferentiatorICPrevScaledInput=0  ExternalReset=none  TrackingMode=off  Kt=1  LimitOutput=off  SatLimitsSource=internal  UpperSaturationLimit=inf  LowerSaturationLimit=-inf  LinearizeAsGain=off  AntiWindupMode=none  Kb=1  POutMin=[]  POutMax=[]  IOutMin=[]  IOutMax=[]  DOutMin=[]  DOutMax=[]  NOutMin=[]  NOutMax=[]  SumOutMin=[]  SumOutMax=[]  SaturationOutMin=[]  SaturationOutMax=[]  PParamMin=[]  PParamMax=[]  IParamMin=[]  IParamMax=[]  DParamMin=[]  DParamMax=[]  NParamMin=[]  NParamMax=[]  KbParamMin=[]  KbParamMax=[]  KtParamMin=[]  KtParamMax=[]  KbOutMin=[]  KbOutMax=[]  KtOutMin=[]  KtOutMax=[]  IntegratorOutMin=[]  IntegratorOutMax=[]  FilterOutMin=[]  FilterOutMax=[]  SumI1OutMin=[]  SumI1OutMax=[]  SumI2OutMin=[]  SumI2OutMax=[]  SumI3OutMin=[]  SumI3OutMax=[]  SumI4OutMin=[]  SumI4OutMax=[]  SumDOutMin=[]  SumDOutMax=[]  DifferentiatorOutMin=[]  DifferentiatorOutMax=[]  FilterDiffOutCoefMin=[]  FilterDiffOutCoefMax=[]  ReciprocalOutMin=[]  ReciprocalOutMax=[]  SumDenOutMin=[]  SumDenOutMax=[]  SumNumOutMin=[]  SumNumOutMax=[]  DivideOutMin=[]  DivideOutMax=[]  UdiffTsProdOutMin=[]  UdiffTsProdOutMax=[]  NTsProdOutMin=[]  NTsProdOutMax=[]  UintegralTsProdOutMin=[]  UintegralTsProdOutMax=[]  UngainTsProdOutMin=[]  UngainTsProdOutMax=[]  IntegratorContinuousStateAttributes=''  IntegratorStateMustResolveToSignalObject=off  IntegratorRTWStateStorageClass=Auto  FilterContinuousStateAttributes=''  FilterStateMustResolveToSignalObject=off  FilterRTWStateStorageClass=Auto  ParallelPVariant=InternalParameters  IdealPVariant=Disabled  IVariant=InternalParameters  DVariant=InternalParameters  IntegratorVariant=Discrete  SatVariant=Disabled  AWVariant=Passthrough  PCopyVariant=Disabled  TRVariant=Disabled  FdbkBlocksVariant=Forward  IdealPFdbkVariant=Disabled  SatFdbkVariant=Disabled  DerivativeFilterVariant=ForwardEulerFilter  NVariant=InternalParameters  NCopyVariant=Disabled  FilterICVariant=InternalICsFilter  IntegratorICVariant=InternalICs  ExternalResetVariant=Disabled  TRSumVariant=Passthrough  SumFdbkVariant=Disabled  SumVariant=Sum_PID  TsampFilterVariant=InternalTs  TsampNgainVariant=Passthrough  TsampIntegralVariant=Passthrough  ExternalSaturationOutDataTypeStr=Inherit: Same as second input  aMode=0
  cfblk4 : DiscreteFir  SampleTime=1
  cfblk5 : Math  Operator=rem
  cfblk6 : Trigonometry
  cfblk7 : Subsystem
  cfblk8 : Subsystem
  cfblk9 : Subsystem
  cfblk2 : Outport
  cfblk15 : Outport  Port=2
  cfblk16 : Outport  Port=3
  cfblk17 : Outport  Port=4
  wires:
  cfblk10/1(cfblk2) -> cfblk9/1(cfblk1)
  cfblk12/1 -> cfblk16/1
  cfblk13/1 -> cfblk8/1(cfblk1)
  cfblk1/1 -> cfblk17/1
  cfblk3/1 -> cfblk10/1(cfblk1)
  cfblk8/1(cfblk2) -> cfblk11/1(cfblk1)
  cfblk8/2(cfblk11) -> cfblk6/1
  cfblk11/1(cfblk2) -> cfblk15/1
  cfblk11/2(cfblk11) -> cfblk5/1
  cfblk4/1 -> cfblk5/2
  cfblk10/2(cfblk16) -> cfblk7/1(cfblk1)
  cfblk7/1(cfblk2) -> cfblk2/1
  cfblk10/3(cfblk17) -> cfblk8/3(cfblk10)
  cfblk14/1 -> cfblk9/2(cfblk7)
  cfblk8/4(cfblk13) -> cfblk4/1
  cfblk9/1(cfblk2) -> cfblk18/1
  cfblk18/1 -> cfblk10/2(cfblk13)
  cfblk9/2(cfblk8) -> cfblk19/1
  cfblk19/1 -> cfblk10/4(cfblk15)
  cfblk5/1 -> cfblk20/1
  cfblk20/1 -> cfblk8/2(cfblk9)
  cfblk6/1 -> cfblk21/1
  cfblk21/1 -> cfblk3/1
  cfblk8/3(cfblk12) -> cfblk22/1
  cfblk22/1 -> cfblk10/3(cfblk14)

== system sampleModel1000/cfblk126 ==
  cfblk1 : Inport
  cfblk11 : Inport  Port=2
  cfblk10 : Subsystem
  cfblk13 : Delay  SampleTime=1
  cfblk3 : slpidlib/PID Controller (2DOF)  Controller=PID  Form=Parallel  TimeDomain=Discrete-time  UseExternalTs=off  SampleTime=1  IntegratorMethod=Forward Euler  FilterMethod=Forward Euler  ControllerParametersSource=internal  P=1  I=1  UseKiTs=off  D=0  N=100  UseFilter=on  b=1  c=1  TunerSelectOption=Transfer Function Based (PID Tuner App)  InitialConditionSource=internal  InitialConditionForIntegrator=0  InitialConditionForFilter=0  DifferentiatorICPrevScaledInput=0  ExternalReset=none  TrackingMode=off  Kt=1  LimitOutput=off  SatLimitsSource=internal  UpperSaturationLimit=inf  LowerSaturationLimit=-inf  LinearizeAsGain=off  AntiWindupMode=none  Kb=1  POutMin=[]  POutMax=[]  IOutMin=[]  IOutMax=[]  DOutMin=[]  DOutMax=[]  NOutMin=[]  NOutMax=[]  bOutMin=[]  bOutMax=[]  cOutMin=[]  cOutMax=[]  SumOutMin=[]  SumOutMax=[]  SaturationOutMin=[]  SaturationOutMax=[]  PParamMin=[]  PParamMax=[]  IParamMin=[]  IParamMax=[]  DParamMin=[]  DParamMax=[]  NParamMin=[]  NParamMax=[]  bParamMin=[]  bParamMax=[]  cParamMin=[]  cParamMax=[]  KbParamMin=[]  KbParamMax=[]  KtParamMin=[]  KtParamMax=[]  KbOutMin=[]  KbOutMax=[]  KtOutMin=[]  KtOutMax=[]  IntegratorOutMin=[]  IntegratorOutMax=[]  FilterOutMin=[]  FilterOutMax=[]  SumI1OutMin=[]  SumI1OutMax=[]  SumI2OutMin=[]  SumI2OutMax=[]  SumI3OutMin=[]  SumI3OutMax=[]  SumI4OutMin=[]  SumI4OutMax=[]  SumDOutMin=[]  SumDOutMax=[]  Sum1OutMin=[]  Sum1OutMax=[]  Sum2OutMin=[]  Sum2OutMax=[]  Sum3OutMin=[]  Sum3OutMax=[]  DifferentiatorOutMin=[]  DifferentiatorOutMax=[]  FilterDiffOutCoefMin=[]  FilterDiffOutCoefMax=[]  ReciprocalOutMin=[]  ReciprocalOutMax=[]  SumDenOutMin=[]  SumDenOutMax=[]  SumNumOutMin=[]  SumNumOutMax=[]  DivideOutMin=[]  DivideOutMax=[]  UdiffTsProdOutMin=[]  UdiffTsProdOutMax=[]  NTsProdOutMin=[]  NTsProdOutMax=[]  UintegralTsProdOutMin=[]  UintegralTsProdOutMax=[]  UngainTsProdOutMin=[]  UngainTsProdOutMax=[]  IntegratorContinuousStateAttributes=''  IntegratorStateMustResolveToSignalObject=off  IntegratorRTWStateStorageClass=Auto  FilterContinuousStateAttributes=''  FilterStateMustResolveToSignalObject=off  FilterRTWStateStorageClass=Auto  ParallelPVariant=InternalParameters  IdealPVariant=Disabled  IVariant=InternalParameters  DVariant=InternalParameters  bVariant=InternalParameters  cVariant=InternalParameters  IntegratorVariant=Discrete  SatVariant=Disabled  AWVariant=Passthrough  PCopyVariant=Disabled  TRVariant=Disabled  FdbkBlocksVariant=Forward  IdealPFdbkVariant=Disabled  SatFdbkVariant=Disabled  DerivativeFilterVariant=ForwardEulerFilter  NVariant=InternalParameters  NCopyVariant=Disabled  FilterICVariant=InternalICsFilter  IntegratorICVariant=InternalICs  ExternalResetVariant=Disabled  TRSumVariant=Passthrough  SumFdbkVariant=Disabled  SumVariant=Sum_PID  TsampFilterVariant=InternalTs  TsampNgainVariant=Passthrough  TsampIntegralVariant=Passthrough  ExternalSaturationOutDataTypeStr=Inherit: Same as second input
      settings: SourceProductBaseCode=SL
  cfblk4 : Sqrt
  cfblk5 : Sqrt
  cfblk6 : Assignment  DiagnosticForDimensions=Warning  IndexOptions=Index vector (dialog)  Indices=1  OutputSizes=1
  cfblk7 : ComplexToMagnitudeAngle
  cfblk8 : Constant  Value=[175423044.447919]  SampleTime=1
  cfblk9 : Constant  Value=[-452867259.274867]  SampleTime=1
  cfblk2 : Outport
  cfblk12 : Outport  Port=2
  wires:
  cfblk8/1 -> cfblk6/1
  cfblk6/1 -> cfblk4/1
  cfblk11/1 -> cfblk5/1
  cfblk7/1 -> cfblk2/1
  cfblk9/1 -> cfblk12/1
  cfblk5/1 -> cfblk6/2
  cfblk1/1 -> cfblk10/1(cfblk1)
  cfblk10/1(cfblk2) -> cfblk7/1
  cfblk4/1 -> cfblk3/1
  cfblk7/2 -> cfblk3/2
  cfblk3/1 -> cfblk13/1
  cfblk13/1 -> cfblk10/2(cfblk7)

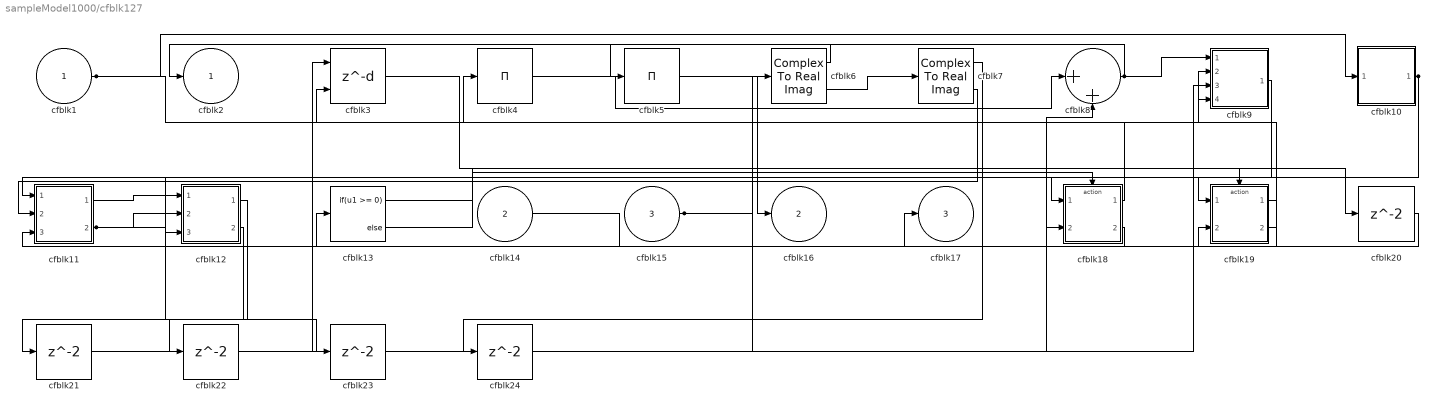
== system sampleModel1000/cfblk127 ==
  cfblk1 : Inport
  cfblk14 : Inport  Port=2
  cfblk15 : Inport  Port=3
  cfblk10 : Subsystem
  cfblk11 : Subsystem
  cfblk12 : Subsystem
  cfblk13 : If  IfExpression=u1 >= 0  SampleTime=1
  cfblk18 : Subsystem  TreatAsAtomicUnit=on
  cfblk19 : Subsystem  TreatAsAtomicUnit=on
  cfblk{20..24} (5 alike) : Delay  SampleTime=1
  cfblk3 : Delay  DelayLengthSource=Input port  SampleTime=1
      settings: InputPortMap=u0,p1
  cfblk4 : Product  Inputs=*
  cfblk5 : Product  Inputs=*
  cfblk6 : ComplexToRealImag
  cfblk7 : ComplexToRealImag
  cfblk8 : Sum  Inputs=|++
  cfblk9 : Subsystem
  cfblk2 : Outport
  cfblk16 : Outport  Port=2
  cfblk17 : Outport  Port=3
  wires:
  cfblk8/1 -> cfblk2/1, cfblk9/1(cfblk1)
  cfblk10/1(cfblk2) -> cfblk18/1(cfblk1), cfblk12/3(cfblk13), cfblk18/2(cfblk15)
  cfblk4/1 -> cfblk8/1
  cfblk19/1(cfblk2) -> cfblk17/1
  cfblk5/1 -> cfblk16/1
  cfblk15/1 -> cfblk19/1(cfblk1), cfblk9/2(cfblk8)
  cfblk14/1 -> cfblk19/2(cfblk14)
  cfblk1/1 -> cfblk10/1(cfblk1), cfblk9/4(cfblk10)
  cfblk19/2(cfblk15) -> cfblk4/1
  cfblk9/1(cfblk2) -> cfblk11/1(cfblk1)
  cfblk18/1(cfblk2) -> cfblk3/2
  cfblk6/1 -> cfblk5/1
  cfblk7/2 -> cfblk11/2(cfblk13)
  cfblk6/2 -> cfblk7/1
  cfblk18/2(cfblk16) -> cfblk11/3(cfblk14)
  cfblk11/1(cfblk2) -> cfblk12/1(cfblk1)
  cfblk11/2(cfblk15) -> cfblk12/2(cfblk12), cfblk23/1
  cfblk13/1 -> cfblk18/Action
  cfblk13/2 -> cfblk19/Action
  cfblk3/1 -> cfblk20/1
  cfblk20/1 -> cfblk13/1
  cfblk12/1(cfblk2) -> cfblk21/1
  cfblk21/1 -> cfblk8/2
  cfblk12/2(cfblk14) -> cfblk22/1
  cfblk22/1 -> cfblk3/1
  cfblk23/1 -> cfblk9/3(cfblk9)
  cfblk7/1 -> cfblk24/1
  cfblk24/1 -> cfblk6/1

== system sampleModel1000/cfblk128 ==
  cfblk1 : Inport
  cfblk13 : Inport  Port=2
  cfblk14 : Inport  Port=3
  cfblk10 : Subsystem
  cfblk11 : Subsystem
  cfblk12 : Subsystem
  cfblk18 : Delay  SampleTime=1
  cfblk19 : Delay  SampleTime=1
  cfblk3 : slpidlib/PID Controller (2DOF)  Controller=PID  Form=Parallel  TimeDomain=Discrete-time  UseExternalTs=off  SampleTime=1  IntegratorMethod=Forward Euler  FilterMethod=Forward Euler  ControllerParametersSource=internal  P=1  I=1  UseKiTs=off  D=0  N=100  UseFilter=on  b=1  c=1  TunerSelectOption=Transfer Function Based (PID Tuner App)  InitialConditionSource=internal  InitialConditionForIntegrator=0  InitialConditionForFilter=0  DifferentiatorICPrevScaledInput=0  ExternalReset=none  TrackingMode=off  Kt=1  LimitOutput=off  SatLimitsSource=internal  UpperSaturationLimit=inf  LowerSaturationLimit=-inf  LinearizeAsGain=off  AntiWindupMode=none  Kb=1  POutMin=[]  POutMax=[]  IOutMin=[]  IOutMax=[]  DOutMin=[]  DOutMax=[]  NOutMin=[]  NOutMax=[]  bOutMin=[]  bOutMax=[]  cOutMin=[]  cOutMax=[]  SumOutMin=[]  SumOutMax=[]  SaturationOutMin=[]  SaturationOutMax=[]  PParamMin=[]  PParamMax=[]  IParamMin=[]  IParamMax=[]  DParamMin=[]  DParamMax=[]  NParamMin=[]  NParamMax=[]  bParamMin=[]  bParamMax=[]  cParamMin=[]  cParamMax=[]  KbParamMin=[]  KbParamMax=[]  KtParamMin=[]  KtParamMax=[]  KbOutMin=[]  KbOutMax=[]  KtOutMin=[]  KtOutMax=[]  IntegratorOutMin=[]  IntegratorOutMax=[]  FilterOutMin=[]  FilterOutMax=[]  SumI1OutMin=[]  SumI1OutMax=[]  SumI2OutMin=[]  SumI2OutMax=[]  SumI3OutMin=[]  SumI3OutMax=[]  SumI4OutMin=[]  SumI4OutMax=[]  SumDOutMin=[]  SumDOutMax=[]  Sum1OutMin=[]  Sum1OutMax=[]  Sum2OutMin=[]  Sum2OutMax=[]  Sum3OutMin=[]  Sum3OutMax=[]  DifferentiatorOutMin=[]  DifferentiatorOutMax=[]  FilterDiffOutCoefMin=[]  FilterDiffOutCoefMax=[]  ReciprocalOutMin=[]  ReciprocalOutMax=[]  SumDenOutMin=[]  SumDenOutMax=[]  SumNumOutMin=[]  SumNumOutMax=[]  DivideOutMin=[]  DivideOutMax=[]  UdiffTsProdOutMin=[]  UdiffTsProdOutMax=[]  NTsProdOutMin=[]  NTsProdOutMax=[]  UintegralTsProdOutMin=[]  UintegralTsProdOutMax=[]  UngainTsProdOutMin=[]  UngainTsProdOutMax=[]  IntegratorContinuousStateAttributes=''  IntegratorStateMustResolveToSignalObject=off  IntegratorRTWStateStorageClass=Auto  FilterContinuousStateAttributes=''  FilterStateMustResolveToSignalObject=off  FilterRTWStateStorageClass=Auto  ParallelPVariant=InternalParameters  IdealPVariant=Disabled  IVariant=InternalParameters  DVariant=InternalParameters  bVariant=InternalParameters  cVariant=InternalParameters  IntegratorVariant=Discrete  SatVariant=Disabled  AWVariant=Passthrough  PCopyVariant=Disabled  TRVariant=Disabled  FdbkBlocksVariant=Forward  IdealPFdbkVariant=Disabled  SatFdbkVariant=Disabled  DerivativeFilterVariant=ForwardEulerFilter  NVariant=InternalParameters  NCopyVariant=Disabled  FilterICVariant=InternalICsFilter  IntegratorICVariant=InternalICs  ExternalResetVariant=Disabled  TRSumVariant=Passthrough  SumFdbkVariant=Disabled  SumVariant=Sum_PID  TsampFilterVariant=InternalTs  TsampNgainVariant=Passthrough  TsampIntegralVariant=Passthrough  ExternalSaturationOutDataTypeStr=Inherit: Same as second input
      settings: SourceProductBaseCode=SL
  cfblk4 : DiscreteIntegrator  ICPrevOutput=DiscIntNeverNeededParam  ICPrevScaledInput=DiscIntNeverNeededParam
  cfblk5 : DiscreteFir  SampleTime=1
  cfblk6 : Polyval  Coefs=[ +2.081618890e-019, -1.441693666e-014, +4.719686976e-010, -8.536869453e-006, +1.621573104e-001, -8.087801117e+001 ]
  cfblk7 : Sum  Inputs=|++
  cfblk8 : Assignment  DiagnosticForDimensions=Warning  IndexOptions=Index vector (dialog)  Indices=1  OutputSizes=1
  cfblk9 : Squeeze
  cfblk2 : Outport
  cfblk15 : Outport  Port=2
  cfblk16 : Outport  Port=3
  cfblk17 : Outport  Port=4
  wires:
  cfblk3/1 -> cfblk7/1
  cfblk6/1 -> cfblk17/1
  cfblk14/1 -> cfblk5/1, cfblk11/1(cfblk1)
  cfblk11/1(cfblk2) -> cfblk12/1(cfblk1)
  cfblk10/1(cfblk2) -> cfblk4/1
  cfblk12/1(cfblk2) -> cfblk6/1
  cfblk7/1 -> cfblk2/1
  cfblk8/1 -> cfblk15/1
  cfblk9/1 -> cfblk7/2
  cfblk13/1 -> cfblk10/1(cfblk1)
  cfblk10/2(cfblk14) -> cfblk16/1, cfblk8/2
  cfblk5/1 -> cfblk9/1
  cfblk1/1 -> cfblk10/2(cfblk11)
  cfblk12/2(cfblk12) -> cfblk8/1
  cfblk4/1 -> cfblk3/1, cfblk18/1, cfblk19/1
  cfblk11/2(cfblk10) -> cfblk3/2
  cfblk18/1 -> cfblk10/3(cfblk12)
  cfblk19/1 -> cfblk10/4(cfblk13)

== system sampleModel1000/cfblk129 ==
  cfblk1 : Inport
  cfblk10 : Constant  Value=[421578713.799676]  SampleTime=1
  cfblk11 : Subsystem
  cfblk12 : Subsystem
  cfblk13 : Subsystem
  cfblk14 : Delay  SampleTime=1
  cfblk15 : Delay  SampleTime=1
  cfblk16 : Delay  SampleTime=1
  cfblk3 : DiscreteIntegrator  ICPrevOutput=DiscIntNeverNeededParam  ICPrevScaledInput=DiscIntNeverNeededParam
  cfblk4 : simulink/Discrete/Tapped Delay  vinit=0.0  samptime=-1  NumDelays=1  DelayOrder=Oldest  includeCurrent=off
  cfblk5 : Rounding
  cfblk6 : UnaryMinus
  cfblk7 : simulink/Math Operations/MinMax Running Resettable  Function=min  vinit=0.0
  cfblk8 : Abs  SaturateOnIntegerOverflow=off
  cfblk9 : Constant  Value=[-37402657.163256]  SampleTime=1
  cfblk2 : Outport
  wires:
  cfblk9/1 -> cfblk2/1
  cfblk3/1 -> cfblk8/1
  cfblk6/1 -> cfblk3/1
  cfblk5/1 -> cfblk13/2(cfblk11)
  cfblk10/1 -> cfblk11/1(cfblk1)
  cfblk12/1(cfblk2) -> cfblk5/1
  cfblk13/1(cfblk2) -> cfblk4/1
  cfblk1/1 -> cfblk12/1(cfblk1)
  cfblk8/1 -> cfblk11/2(cfblk11)
  cfblk7/1 -> cfblk11/3(cfblk12)
  cfblk13/2(cfblk12) -> cfblk6/1
  cfblk13/3(cfblk13) -> cfblk7/1
  cfblk13/4(cfblk14) -> cfblk7/2
  cfblk4/1 -> cfblk14/1
  cfblk14/1 -> cfblk13/1(cfblk1)
  cfblk11/1(cfblk2) -> cfblk15/1
  cfblk15/1 -> cfblk12/2(cfblk8)
  cfblk11/2(cfblk13) -> cfblk16/1
  cfblk16/1 -> cfblk12/3(cfblk9)

== system sampleModel1000/cfblk130 ==
  cfblk1 : Inport
  cfblk3 : Delay  DelayLengthSource=Input port  SampleTime=1
      settings: InputPortMap=u0,p1
  cfblk4 : Subsystem
  cfblk5 : Subsystem
  cfblk6 : Subsystem
  cfblk8 : Delay  SampleTime=1
  cfblk9 : Delay  SampleTime=1
  cfblk2 : Outport
  cfblk7 : Outport  Port=2
  wires:
  cfblk1/1 -> cfblk3/1, cfblk6/2(cfblk11), cfblk3/2, cfblk5/1(cfblk1)
  cfblk3/1 -> cfblk7/1, cfblk5/2(cfblk9), cfblk6/4(cfblk13)
  cfblk4/1(cfblk2) -> cfblk2/1, cfblk8/1, cfblk9/1
  cfblk5/1(cfblk2) -> cfblk6/1(cfblk1), cfblk6/5(cfblk14)
  cfblk6/1(cfblk2) -> cfblk4/1(cfblk1)
  cfblk8/1 -> cfblk5/3(cfblk10)
  cfblk9/1 -> cfblk6/3(cfblk12)

== system sampleModel1000/cfblk131 ==
  cfblk1 : Inport
  cfblk10 : Subsystem  TreatAsAtomicUnit=on
  cfblk{3,11..17} (8 alike) : Delay  SampleTime=1
  cfblk4 : Product
  cfblk5 : Subsystem
  cfblk6 : Subsystem
  cfblk7 : If  IfExpression=u1 >= 0  SampleTime=1
  cfblk9 : Subsystem  TreatAsAtomicUnit=on
  cfblk2 : Outport
  cfblk8 : Outport  Port=2
  wires:
  cfblk6/1(cfblk2) -> cfblk3/1, cfblk4/1, cfblk15/1
  cfblk10/1(cfblk2) -> cfblk12/1, cfblk13/1
  cfblk9/1(cfblk2) -> cfblk6/2(cfblk15)
  cfblk3/1 -> cfblk2/1, cfblk11/1, cfblk14/1
  cfblk1/1 -> cfblk5/1(cfblk1)
  cfblk5/1(cfblk2) -> cfblk9/1(cfblk1)
  cfblk5/2(cfblk10) -> cfblk10/1(cfblk1), cfblk4/2
  cfblk9/3(cfblk15) -> cfblk8/1
  cfblk7/1 -> cfblk9/Action
  cfblk7/2 -> cfblk10/Action
  cfblk11/1 -> cfblk10/2(cfblk9)
  cfblk12/1 -> cfblk7/1
  cfblk13/1 -> cfblk5/3(cfblk9)
  cfblk14/1 -> cfblk9/3(cfblk13)
  cfblk15/1 -> cfblk9/2(cfblk12)
  cfblk4/1 -> cfblk16/1
  cfblk16/1 -> cfblk6/1(cfblk1)
  cfblk9/2(cfblk14) -> cfblk17/1
  cfblk17/1 -> cfblk5/2(cfblk8)

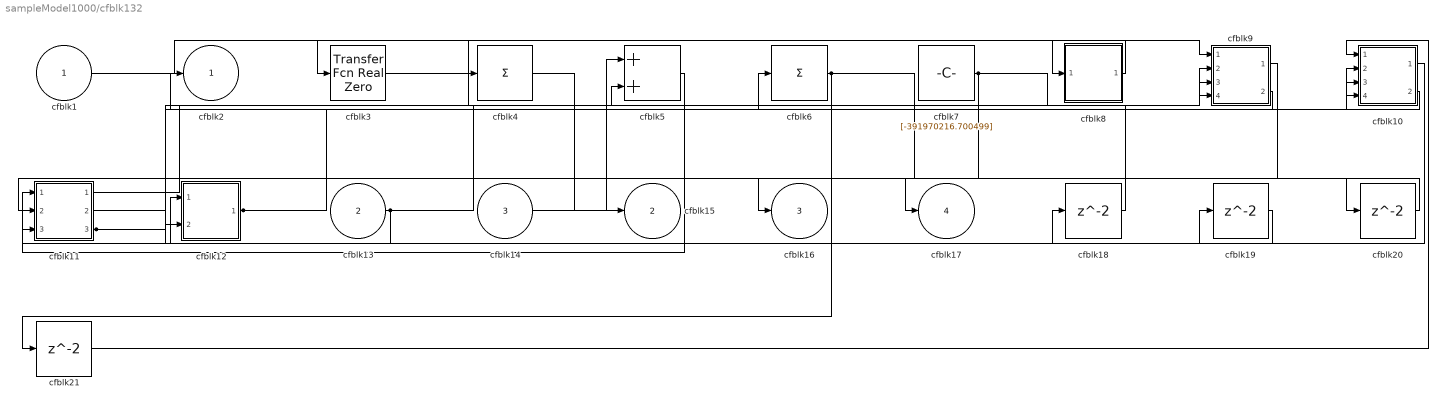
== system sampleModel1000/cfblk132 ==
  cfblk1 : Inport
  cfblk13 : Inport  Port=2
  cfblk14 : Inport  Port=3
  cfblk10 : Subsystem
  cfblk11 : Subsystem
  cfblk12 : Subsystem
  cfblk{18..21} (4 alike) : Delay  SampleTime=1
  cfblk3 : simulink/Discrete/Transfer Fcn Real Zero  ZeroZ=0.75  ICPrevInput=0.0  DoSatur=off
      settings: SourceProductBaseCode=SL
  cfblk4 : Sum  Inputs=+
  cfblk5 : Sum
  cfblk6 : Sum  Inputs=+
  cfblk7 : Constant  Value=[-391970216.700499]  SampleTime=1
  cfblk8 : Subsystem
  cfblk9 : Subsystem
  cfblk2 : Outport
  cfblk15 : Outport  Port=2
  cfblk16 : Outport  Port=3
  cfblk17 : Outport  Port=4
  wires:
  cfblk4/1 -> cfblk15/1
  cfblk11/1(cfblk2) -> cfblk9/1(cfblk1)
  cfblk14/1 -> cfblk5/1
  cfblk13/1 -> cfblk12/1(cfblk1), cfblk9/4(cfblk16)
  cfblk8/1(cfblk2) -> cfblk3/1
  cfblk5/1 -> cfblk11/1(cfblk1)
  cfblk7/1 -> cfblk12/2(cfblk11), cfblk9/3(cfblk15)
  cfblk12/1(cfblk2) -> cfblk16/1, cfblk10/2(cfblk14), cfblk10/3(cfblk15)
  cfblk6/1 -> cfblk20/1, cfblk21/1
  cfblk11/2(cfblk11) -> cfblk9/2(cfblk14)
  cfblk3/1 -> cfblk4/1
  cfblk11/3(cfblk12) -> cfblk10/4(cfblk16), cfblk18/1
  cfblk9/1(cfblk2) -> cfblk17/1
  cfblk1/1 -> cfblk8/1(cfblk1)
  cfblk10/2(cfblk17) -> cfblk6/1
  cfblk9/2(cfblk17) -> cfblk2/1
  cfblk18/1 -> cfblk5/2
  cfblk10/1(cfblk2) -> cfblk19/1
  cfblk19/1 -> cfblk11/3(cfblk10)
  cfblk20/1 -> cfblk11/2(cfblk9)
  cfblk21/1 -> cfblk10/1(cfblk1)

== system sampleModel1000/cfblk133 ==
  cfblk1 : Inport
  cfblk10 : Subsystem
  cfblk{11..14} (4 alike) : Delay  SampleTime=1
  cfblk3 : DiscreteFilter  SampleTime=1
  cfblk4 : DiscreteIntegrator  ICPrevOutput=DiscIntNeverNeededParam  ICPrevScaledInput=DiscIntNeverNeededParam
  cfblk5 : simulink/Discrete/Tapped Delay  vinit=0.0  samptime=-1  NumDelays=1  DelayOrder=Oldest  includeCurrent=off
  cfblk6 : Abs  SaturateOnIntegerOverflow=off
  cfblk7 : Bias  Bias=[-186956224.200085]  SaturateOnIntegerOverflow=off
  cfblk8 : Constant  Value=[73449431.824764]  SampleTime=1
  cfblk9 : Subsystem
  cfblk2 : Outport
  wires:
  cfblk6/1 -> cfblk5/1
  cfblk4/1 -> cfblk7/1
  cfblk8/1 -> cfblk9/1(cfblk1)
  cfblk7/1 -> cfblk9/2(cfblk10)
  cfblk3/1 -> cfblk4/1
  cfblk9/2(cfblk14) -> cfblk6/1
  cfblk1/1 -> cfblk2/1
  cfblk5/1 -> cfblk10/1(cfblk1)
  cfblk9/1(cfblk2) -> cfblk11/1
  cfblk11/1 -> cfblk3/1
  cfblk10/1(cfblk2) -> cfblk12/1
  cfblk12/1 -> cfblk9/3(cfblk11)
  cfblk10/2(cfblk9) -> cfblk13/1
  cfblk13/1 -> cfblk9/4(cfblk12)
  cfblk10/3(cfblk10) -> cfblk14/1
  cfblk14/1 -> cfblk9/5(cfblk13)
